simulink model "DSM_MOD8_HDL"  (R2017b)
settings: Solver=FixedStepDiscrete  StartTime=0.0  StopTime=N/Fs  RelTol=1e-3
undefined symbols (not defined in the file or in its folder): a, b, c, g
settings Model: Creator=o_cotte  LastModifiedBy=o_cotte
settings DataIOCC: LimitDataPoints=on  SaveFormat=Array  SignalLoggingSaveFormat=ModelDataLogs
settings OptimizationCC: BlockReduction=off  BooleanDataType=off  ConditionallyExecuteInputs=off  DefaultParameterBehavior=Inlined  LifeSpan=inf
settings DebuggingCC: AlgebraicLoopMsg=error  SaveWithParameterizedLinksMsg=none  UnderspecifiedInitializationDetection=Classic  MergeDetectMultiDrivingBlocksExec=none  SignalResolutionControl=TryResolveAllWithWarning  MultiTaskDSMMsg=warning  MultiTaskCondExecSysMsg=none  SFUnexpectedBacktrackingDiag=warning  SFNoUnconditionalDefaultTransitionDiag=warning  SFExecutionAtInitializationDiag=none
settings HardwareCC: ProdBitPerPointer=32  ProdBitPerSizeT=32  ProdBitPerPtrDiffT=32  ProdLargestAtomicFloat=None  ProdIntDivRoundTo=Undefined  ProdEndianess=Unspecified  ProdWordSize=32  ProdHWDeviceType=ASIC/FPGA->ASIC/FPGA  TargetBitPerPointer=64  TargetBitPerSizeT=64  TargetBitPerPtrDiffT=64  TargetLongLongMode=on  TargetIntDivRoundTo=Zero  TargetEndianess=LittleEndian  TargetWordSize=64  TargetHWDeviceType=MATLAB Host  ProdEqTarget=off
settings ModelReferenceCC: PropagateSignalLabelsOutOfModel=off
settings CodeAppCC: StateflowObjectComments=on
settings GRTTargetCC: TargetLangStandard=C89/C90 (ANSI)  GeneratePreprocessorConditionals=Disable all
settings ConfigComp: CovMetricSettings=dw  CovHtmlReporting=on  CovSaveCumulativeToWorkspaceVar=on  CovSaveSingleToWorkspaceVar=on  CovExternalEMLEnable=off

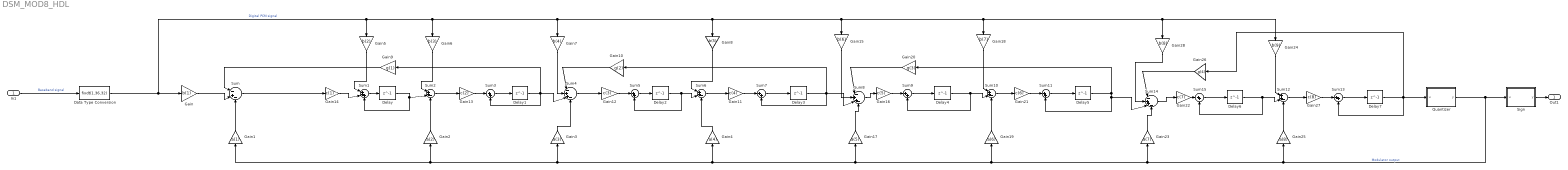
== system DSM_MOD8_HDL ==
  In1 : Inport
  Data Type Conversion : DataTypeConversion  OutDataTypeStr=fixdt(1,36,32)
  Delay{,1..7} (8 alike) : Delay  DelayLength=1  InitialCondition=0
  Gain : Gain  Gain=b(1)  OutDataTypeStr=Inherit: Same as input  ParamDataTypeStr=Inherit: Same as input  LockScale=on
  Gain1 : Gain  Gain=a(1)  OutDataTypeStr=Inherit: Same as input
  Gain10 : Gain  Gain=g(2)  OutDataTypeStr=Inherit: Same as input  ParamDataTypeStr=Inherit: Same as input  LockScale=on
  Gain11 : Gain  Gain=c(4)  OutDataTypeStr=Inherit: Same as input  ParamDataTypeStr=Inherit: Same as input  LockScale=on
  Gain12 : Gain  Gain=c(3)  OutDataTypeStr=Inherit: Same as input  ParamDataTypeStr=Inherit: Same as input  LockScale=on
  Gain13 : Gain  Gain=c(2)  OutDataTypeStr=Inherit: Same as input  ParamDataTypeStr=Inherit: Same as input  LockScale=on
  Gain14 : Gain  Gain=c(1)  OutDataTypeStr=Inherit: Same as input  ParamDataTypeStr=Inherit: Same as input  LockScale=on
  Gain15 : Gain  Gain=b(6)  OutDataTypeStr=Inherit: Same as input  ParamDataTypeStr=Inherit: Same as input  LockScale=on
  Gain16 : Gain  Gain=c(5)  OutDataTypeStr=Inherit: Same as input  ParamDataTypeStr=Inherit: Same as input  LockScale=on
  Gain17 : Gain  Gain=a(5)  OutDataTypeStr=Inherit: Same as input
  Gain18 : Gain  Gain=b(7)  OutDataTypeStr=Inherit: Same as input  ParamDataTypeStr=Inherit: Same as input  LockScale=on
  Gain19 : Gain  Gain=a(6)  OutDataTypeStr=Inherit: Same as input
  Gain2 : Gain  Gain=a(2)  OutDataTypeStr=Inherit: Same as input
  Gain20 : Gain  Gain=g(3)  OutDataTypeStr=Inherit: Same as input  ParamDataTypeStr=Inherit: Same as input  LockScale=on
  Gain21 : Gain  Gain=c(6)  OutDataTypeStr=Inherit: Same as input  ParamDataTypeStr=Inherit: Same as input  LockScale=on
  Gain22 : Gain  Gain=c(7)  OutDataTypeStr=Inherit: Same as input  ParamDataTypeStr=Inherit: Same as input  LockScale=on
  Gain23 : Gain  Gain=a(7)  OutDataTypeStr=Inherit: Same as input
  Gain24 : Gain  Gain=b(9)  OutDataTypeStr=Inherit: Same as input  ParamDataTypeStr=Inherit: Same as input  LockScale=on
  Gain25 : Gain  Gain=a(8)  OutDataTypeStr=Inherit: Same as input
  Gain26 : Gain  Gain=g(4)  OutDataTypeStr=Inherit: Same as input  ParamDataTypeStr=Inherit: Same as input  LockScale=on
  Gain27 : Gain  Gain=c(8)  OutDataTypeStr=Inherit: Same as input  ParamDataTypeStr=Inherit: Same as input  LockScale=on
  Gain28 : Gain  Gain=b(8)  OutDataTypeStr=Inherit: Same as input  ParamDataTypeStr=Inherit: Same as input  LockScale=on
  Gain3 : Gain  Gain=a(3)  OutDataTypeStr=Inherit: Same as input
  Gain4 : Gain  Gain=a(4)  OutDataTypeStr=Inherit: Same as input
  Gain5 : Gain  Gain=b(2)  OutDataTypeStr=Inherit: Same as input  ParamDataTypeStr=Inherit: Same as input  LockScale=on
  Gain6 : Gain  Gain=b(3)  OutDataTypeStr=Inherit: Same as input  ParamDataTypeStr=Inherit: Same as input  LockScale=on
  Gain7 : Gain  Gain=b(4)  OutDataTypeStr=Inherit: Same as input  ParamDataTypeStr=Inherit: Same as input  LockScale=on
  Gain8 : Gain  Gain=b(5)  OutDataTypeStr=Inherit: Same as input  ParamDataTypeStr=Inherit: Same as input  LockScale=on
  Gain9 : Gain  Gain=g(1)  OutDataTypeStr=Inherit: Same as input  ParamDataTypeStr=Inherit: Same as input  LockScale=on
  Quantizer : MATLAB Function  TreatAsAtomicUnit=on
  Sign : MATLAB Function  TreatAsAtomicUnit=on
  Sum : Sum  Inputs=|-+-  OutDataTypeStr=Inherit: Same as accumulator  LockScale=on
  Sum1 : Sum  Inputs=|+++  OutDataTypeStr=Inherit: Same as accumulator  LockScale=on
  Sum{2,6,10,12} (4 alike) : Sum  Inputs=|++-  OutDataTypeStr=Inherit: Same as accumulator  LockScale=on
  Sum{3,5,7,9,11,13,15} (7 alike) : Sum  Inputs=|++  OutDataTypeStr=Inherit: Same as accumulator  LockScale=on
  Sum14 : Sum  Inputs=|-++-  OutDataTypeStr=Inherit: Same as accumulator  LockScale=on
  Sum4 : Sum  Inputs=|-++-  OutDataTypeStr=Inherit: Same as accumulator  LockScale=on
  Sum8 : Sum  Inputs=|-++-  OutDataTypeStr=Inherit: Same as accumulator  LockScale=on
  Out1 : Outport
  wires:
  Sum/1 -> Gain14/1
  Gain/1 -> Sum/2
  In1/1 -> Data Type Conversion/1  "Baseband signal"
  Gain1/1 -> Sum/3
  Gain2/1 -> Sum2/3
  Gain3/1 -> Sum4/4
  Gain4/1 -> Sum6/3
  Sum3/1 -> Delay1/1
  Sum7/1 -> Delay3/1
  Sum1/1 -> Delay/1
  Delay1/1 -> Sum3/2, Gain9/1, Sum4/3
  Sum5/1 -> Delay2/1
  Gain5/1 -> Sum1/1
  Sum2/1 -> Gain13/1
  Gain6/1 -> Sum2/1
  Gain7/1 -> Sum4/2
  Gain8/1 -> Sum6/1
  Sum6/1 -> Gain11/1
  Sum4/1 -> Gain12/1
  Delay/1 -> Sum1/3, Sum2/2
  Delay2/1 -> Sum5/2, Sum6/2
  Gain10/1 -> Sum4/1
  Delay3/1 -> Sum8/3, Sum7/2, Gain10/1
  Gain9/1 -> Sum/1
  Gain11/1 -> Sum7/1
  Gain12/1 -> Sum5/1
  Gain13/1 -> Sum3/1
  Gain14/1 -> Sum1/2
  Gain15/1 -> Sum8/2
  Sum8/1 -> Gain16/1
  Gain17/1 -> Sum8/4
  Gain16/1 -> Sum9/1
  Delay4/1 -> Sum9/2, Sum10/2
  Sum9/1 -> Delay4/1
  Gain18/1 -> Sum10/1
  Gain19/1 -> Sum10/3
  Sum10/1 -> Gain21/1
  Sum11/1 -> Delay5/1
  Gain20/1 -> Sum8/1
  Gain21/1 -> Sum11/1
  Sum14/1 -> Gain22/1
  Gain23/1 -> Sum14/4
  Gain27/1 -> Sum13/1
  Gain26/1 -> Sum14/1
  Sum13/1 -> Delay7/1
  Quantizer/1(y) -> Gain25/1, Gain1/1, Gain2/1, Gain3/1, Gain4/1, Gain17/1, Gain19/1, Gain23/1, Sign/1(u)  "Modulator output"
  Sum12/1 -> Gain27/1
  Sum15/1 -> Delay6/1
  Data Type Conversion/1 -> Gain5/1, Gain8/1, Gain18/1, Gain28/1, Gain24/1, Gain15/1, Gain7/1, Gain6/1, Gain/1  "Digital PCM signal"
  Gain25/1 -> Sum12/3
  Delay6/1 -> Sum15/2, Sum12/2
  Delay5/1 -> Sum14/3, Sum11/2, Gain20/1
  Gain22/1 -> Sum15/1
  Delay7/1 -> Quantizer/1(u), Sum13/2, Gain26/1
  Gain24/1 -> Sum12/1
  Gain28/1 -> Sum14/2
  Sign/1(y) -> Out1/1

== matlab function DSM_MOD8_HDL/Sign ==
  data: u input; y output
function y = fcn(u)
%#codegen
if u < 0
    y = fi(-1,1,2,0);
else
    y = fi(1,1,2,0);
end

== matlab function DSM_MOD8_HDL/Quantizer ==
  data: u input; y output
function y = fcn(u)
%#codegen
if u < 0
    y = fi(-1,1,36,32);
else
    y = fi(1,1,36,32);
end
